simulink library "Rail_UL"  (R2019a)
settings: Solver=VariableStepAuto  StartTime=0.0  StopTime=10.0  RelTol=1e-3
settings Model: Creator=jbore  LastModifiedBy=jbore

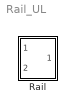
== system Rail_UL ==
  Rail : Subsystem  mask{z_r=0, a_out=0}
      mask prompts: z_r "Rail length [m]"; a_out "Held output value"
      mask DialogControl DescGroupVar Prompt: Launch Rail Library
      mask DialogControl DescTextVar Prompt: This block holds the output to specified value until vehicle is clear of launch rail.
      mask Display:
      | patch([0 1 1 0], [0 0 1 1],[.8 1 1])
      | 
      | port_label('input',1,'\fontname{Cambria Math}In','texmode','on')
      | port_label('input',2,'\fontname{Cambria Math}Alt','texmode','on')
      | 
      | port_label('output',1,'\fontname{Cambria Math}Out','texmode','on')

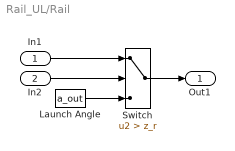
== system Rail_UL/Rail ==
  In1 : Inport
  In2 : Inport  Port=2
  Launch Angle : Constant  Value=a_out
  Switch : Switch  Criteria=u2 > Threshold  Threshold=z_r
  Out1 : Outport
  wires:
  Launch Angle/1 -> Switch/3
  In2/1 -> Switch/2
  In1/1 -> Switch/1
  Switch/1 -> Out1/1
